simulink model "W3_Prob3"  (R2020b)
settings: Solver=ode45  StartTime=0.0  StopTime=2.0  RelTol=1e-3
undefined symbols (not defined in the file or in its folder): b1, b2, K, k1, k2, m1, m2
settings Model: DataDictionary=W3_Prob3.sldd  Creator=shoun  LastModifiedBy=shoun

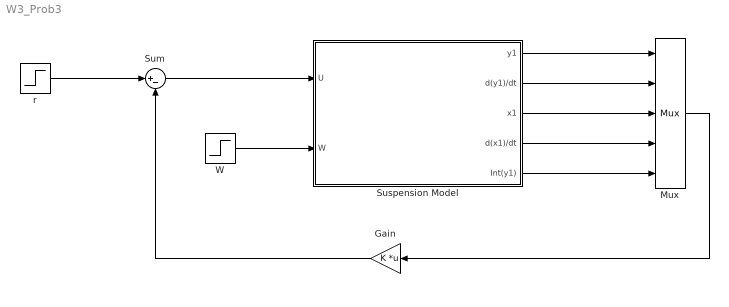
== system W3_Prob3 ==
  Gain : Gain  Gain=K  Multiplication=Matrix(K*u)
  Mux : Mux  Inputs=5
  Sum : Sum  Inputs=|+-
  Suspension Model : Subsystem
  W : Step  Time=0  After=-1  SampleTime=0
  r : Step  Time=0  After=0  SampleTime=0
  wires:
  r/1 -> Sum/1
  Sum/1 -> Suspension Model/1(U)
  W/1 -> Suspension Model/2(W)
  Gain/1 -> Sum/2
  Suspension Model/1(y1) -> Mux/1
  Suspension Model/2(d(y1)/dt) -> Mux/2
  Suspension Model/3(x1) -> Mux/3
  Suspension Model/4(d(x1)/dt) -> Mux/4
  Suspension Model/5(Int(y1)) -> Mux/5
  Mux/1 -> Gain/1

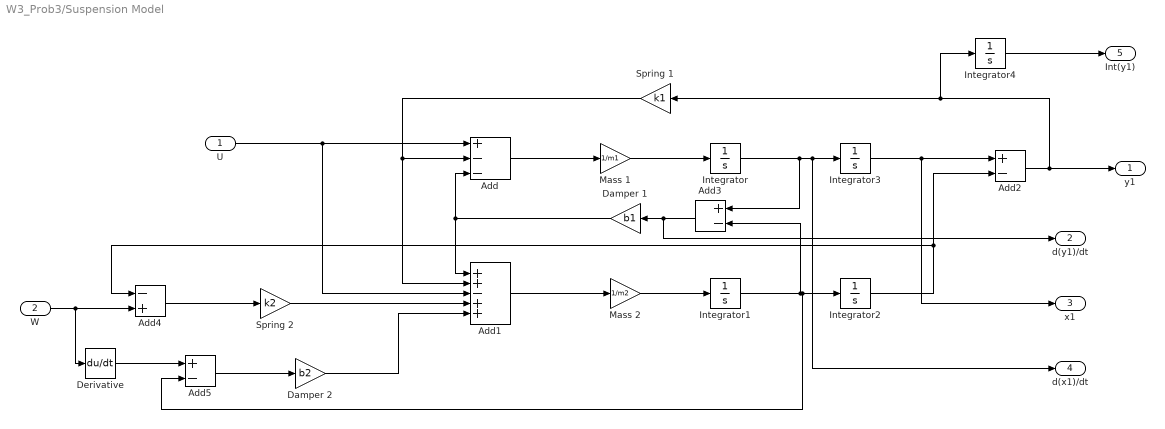
== system W3_Prob3/Suspension Model ==
  U : Inport
  W : Inport  Port=2
  Add : Sum  Inputs=+--
  Add1 : Sum  Inputs=++-++
  Add2 : Sum  Inputs=+-
  Add3 : Sum  Inputs=+-
  Add4 : Sum  Inputs=-+
  Add5 : Sum  Inputs=+-
  Damper 1 : Gain  Gain=b1
  Damper 2 : Gain  Gain=b2
  Derivative : Derivative
  Integrator{,1..4} (5 alike) : Integrator
  Mass 1 : Gain  Gain=1/m1
  Mass 2 : Gain  Gain=1/m2
  Spring 1 : Gain  Gain=k1
  Spring 2 : Gain  Gain=k2
  y1 : Outport
  d(y1)/dt : Outport  Port=2
  x1 : Outport  Port=3
  d(x1)/dt : Outport  Port=4
  Int(y1) : Outport  Port=5
  wires:
  U/1 -> Add1/3, Add/1
  W/1 -> Derivative/1, Add4/2
  Add3/1 -> d(y1)/dt/1, Damper 1/1
  Integrator/1 -> Add3/1, d(x1)/dt/1, Integrator3/1
  Integrator1/1 -> Add3/2, Add5/2, Integrator2/1
  Mass 1/1 -> Integrator/1
  Spring 1/1 -> Add/2, Add1/2
  Add1/1 -> Mass 2/1
  Integrator4/1 -> Int(y1)/1
  Damper 2/1 -> Add1/5
  Add/1 -> Mass 1/1
  Spring 2/1 -> Add1/4
  Integrator2/1 -> Add4/1, Add2/2
  Add5/1 -> Damper 2/1
  Damper 1/1 -> Add1/1, Add/3
  Add2/1 -> y1/1, Integrator4/1, Spring 1/1
  Add4/1 -> Spring 2/1
  Integrator3/1 -> x1/1, Add2/1
  Derivative/1 -> Add5/1
  Mass 2/1 -> Integrator1/1
